simulink model "Aufgabe3_sim"  (R2023b)
settings: Solver=VariableStepAuto  StartTime=0.0  StopTime=1  RelTol=1e-3
values from neighbouring files (symbols this model uses):
  ci = 0.01    [Aufgabe3_param.m]
  cy = 1    [Aufgabe3_param.m]
  high_lim = 0.005    [Aufgabe3_param.m]
  init_pos = -0.001    [Aufgabe3_param.m]
  Kr = 4000    [Aufgabe3_param.m]
  L = 0.1    [Aufgabe3_param.m]
  low_lim = -0.05    [Aufgabe3_param.m]
  m = 10e-3    (= 0.01)    [Aufgabe3_param.m]
  op_lim = 6    [Aufgabe3_param.m]
  R = 5    [Aufgabe3_param.m]
  Tv = Tv_array(count)    [Aufgabe3_param.m]
settings Model: Creator=rouven  LastModifiedBy=rouven

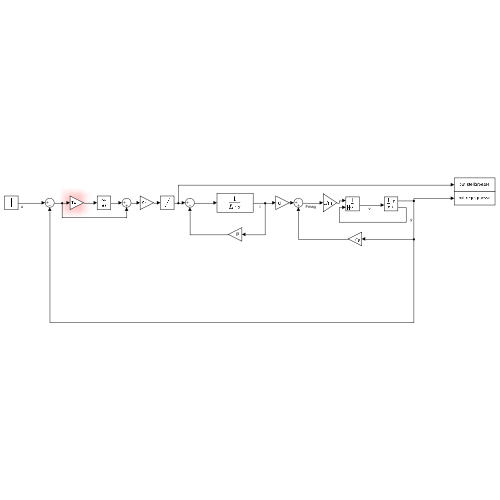
[thumbnail: Simulink's stored preview of the top-level diagram]
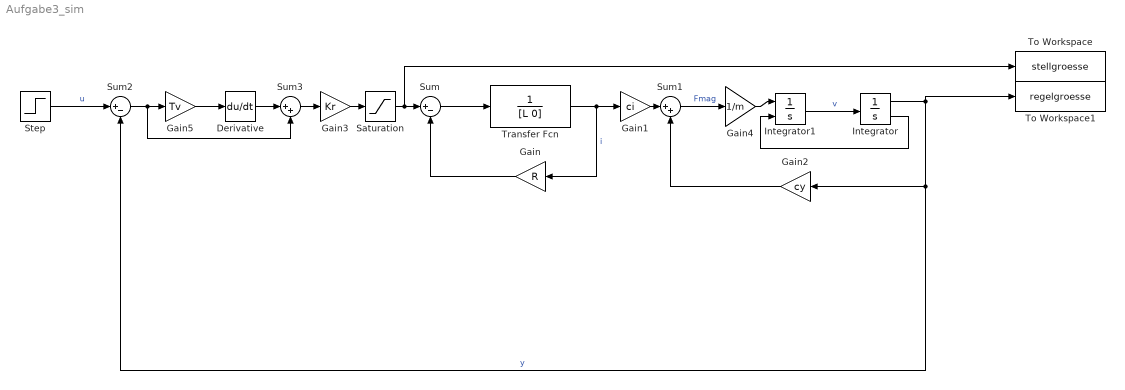
== system Aufgabe3_sim ==
  Derivative : Derivative
  Gain : Gain  Gain=R
  Gain1 : Gain  Gain=ci
  Gain2 : Gain  Gain=cy
  Gain3 : Gain  Gain=Kr
  Gain4 : Gain  Gain=1/m
  Gain5 : Gain  Gain=Tv
  Integrator : Integrator  InitialCondition=init_pos  LimitOutput=on  UpperSaturationLimit=high_lim  LowerSaturationLimit=low_lim  ShowSaturationPort=on
  Integrator1 : Integrator  ExternalReset=either
  Saturation : Saturate  UpperLimit=op_lim  LowerLimit=-op_lim
  Step : Step  Time=0  After=0  SampleTime=0
  Sum : Sum  Inputs=|+-
  Sum1 : Sum  Inputs=|++
  Sum2 : Sum  Inputs=|+-
  Sum3 : Sum  Inputs=|++
  To Workspace : ToWorkspace  VariableName=stellgroesse  SaveFormat=Timeseries  SampleTime=-1
  To Workspace1 : ToWorkspace  VariableName=regelgroesse  SaveFormat=Timeseries  SampleTime=-1
  Transfer Fcn : TransferFcn  Denominator=[L 0]
  wires:
  Sum/1 -> Transfer Fcn/1
  Gain/1 -> Sum/2
  Transfer Fcn/1 -> Gain/1, Gain1/1  "i"
  Gain1/1 -> Sum1/1
  Sum1/1 -> Gain4/1  "Fmag"
  Integrator1/1 -> Integrator/1  "v"
  Integrator/1 -> Gain2/1, Sum2/2, To Workspace1/1  "y"
  Gain2/1 -> Sum1/2
  Saturation/1 -> To Workspace/1, Sum/1
  Gain3/1 -> Saturation/1
  Step/1 -> Sum2/1  "u"
  Gain4/1 -> Integrator1/1
  Integrator/2 -> Integrator1/2
  Gain5/1 -> Derivative/1
  Derivative/1 -> Sum3/1
  Sum2/1 -> Sum3/2, Gain5/1
  Sum3/1 -> Gain3/1
